simulink model "boost_converter_example"  (R2025a)
settings: Solver=FixedStepAuto  StartTime=0.0  StopTime=Tfin  FixedStep=Ts  RelTol=1e-3
values from neighbouring files (symbols this model uses):
  static_gain = 1.76    [experiment_setup_simulink.m]
  time_constant = 0.5    [experiment_setup_simulink.m]
  u0 = 0    [experiment_setup_simulink.m]    (also in generare_subiect_norocos_TOATE_2024.m = 30+5*rand(1); ordin1_treapta.m = mean(u(i1:i2)); ordin2_treapta.m = mean(u(i1:i2)))
  ust = 2    [experiment_setup_simulink.m]    (also in generare_subiect_norocos_TOATE_2024.m = u0+20*rand(1); master_tapes_ord2_imp_reg_mod.m = mean(u(i1:i2)); ordin1_treapta.m = mean(u(j1:j2)); ordin2_treapta.m = mean(u(j1:j2)))
  whtn_pow_in = 1e-5    (= 1e-05)    [experiment_setup_simulink.m]
  whtn_pow_out = 1e-6    (= 1e-06)    [experiment_setup_simulink.m]
  whtn_seed_in = 23341    [experiment_setup_simulink.m]
  whtn_seed_out = 23342    [experiment_setup_simulink.m]
  whtn_Ts_in = Ts    (= 0.01)    [experiment_setup_simulink.m]
  whtn_Ts_out = Ts    (= 0.01)    [experiment_setup_simulink.m]
  x0 = -0.5    [experiment_setup_simulink.m]
libraries: simulink x3
settings Model: Creator=mircea  LastModifiedBy=mircea

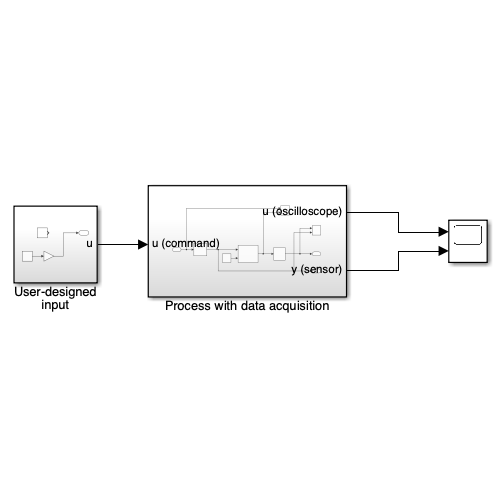
[thumbnail: Simulink's stored preview of the top-level diagram]
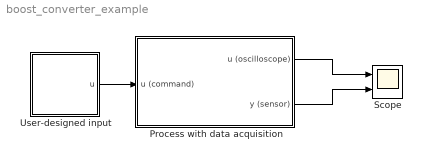
== system boost_converter_example ==
  Process with data acquisition : Subsystem
  Scope : Scope  NumInputPorts=2
      settings: ActiveDisplayYMinimum=-3.990234375  ActiveDisplayYMaximum=5.130859375
  User-designed input : Subsystem
  wires:
  Process with data acquisition/1(u (oscilloscope)) -> Scope/1
  Process with data acquisition/2(y (sensor)) -> Scope/2
  User-designed input/1(u) -> Process with data acquisition/1(u (command))

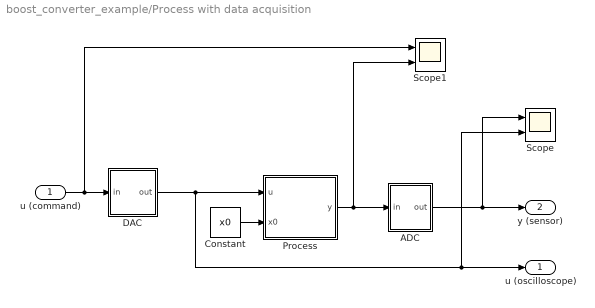
== system boost_converter_example/Process with data acquisition ==
  u (command) : Inport
  ADC : Subsystem
  Constant : Constant  Value=x0
  DAC : Subsystem
  Process : Subsystem
  Scope : Scope  NumInputPorts=2
      settings: ActiveDisplayYMinimum=-1.328125  ActiveDisplayYMaximum=1.328125
  Scope1 : Scope  NumInputPorts=2
      settings: ActiveDisplayYMinimum=-1.328125  ActiveDisplayYMaximum=1.328125  DataLoggingVariableName=ScopeData2
  u (oscilloscope) : Outport
  y (sensor) : Outport  Port=2
  wires:
  Constant/1 -> Process/2(x0)
  u (command)/1 -> Scope1/1, DAC/1(in)
  Process/1(y) -> Scope1/2, ADC/1(in)
  ADC/1(out) -> Scope/1, y (sensor)/1
  DAC/1(out) -> Scope/2, u (oscilloscope)/1, Process/1(u)

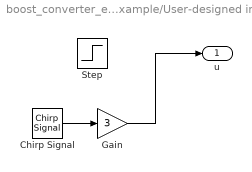
== system boost_converter_example/User-designed input ==
  Chirp Signal : simulink/Sources/Chirp Signal  f1=0.01  T=80  f2=15
  Gain : Gain  Gain=3
  Step : Step  Before=u0  After=ust  SampleTime=0
  u : Outport
  wires:
  Chirp Signal/1 -> Gain/1
  Gain/1 -> u/1

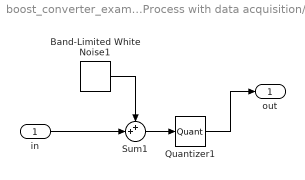
== system boost_converter_example/Process with data acquisition/ADC ==
  in : Inport
  Band-Limited White Noise1 : simulink/Sources/Band-Limited White Noise  Cov=[whtn_pow_out]  Ts=whtn_Ts_out  seed=[whtn_seed_out]
  Quantizer1 : Quantizer  QuantizationInterval=q_out
  Sum1 : Sum  Inputs=++|
  out : Outport
  wires:
  Quantizer1/1 -> out/1
  Sum1/1 -> Quantizer1/1
  in/1 -> Sum1/2
  Band-Limited White Noise1/1 -> Sum1/1

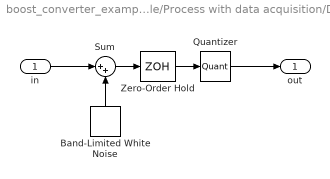
== system boost_converter_example/Process with data acquisition/DAC ==
  in : Inport
  Band-Limited White Noise : simulink/Sources/Band-Limited White Noise  Cov=[whtn_pow_in]  Ts=whtn_Ts_in  seed=[whtn_seed_in]
  Quantizer : Quantizer  QuantizationInterval=q_in
  Sum : Sum  Inputs=|++
  Zero-Order Hold : ZeroOrderHold  SampleTime=-1
  out : Outport
  wires:
  Quantizer/1 -> out/1
  Sum/1 -> Zero-Order Hold/1
  in/1 -> Sum/1
  Band-Limited White Noise/1 -> Sum/2
  Zero-Order Hold/1 -> Quantizer/1

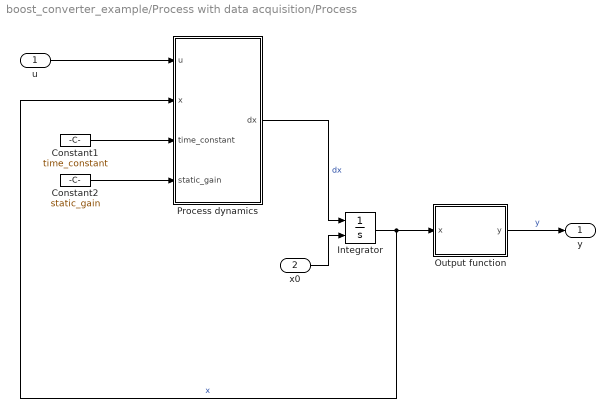
== system boost_converter_example/Process with data acquisition/Process ==
  u : Inport
  x0 : Inport  Port=2
  Constant1 : Constant  Value=time_constant
  Constant2 : Constant  Value=static_gain
  Integrator : Integrator  InitialConditionSource=external
  Output function : MATLAB Function  TreatAsAtomicUnit=on
  Process dynamics : MATLAB Function  TreatAsAtomicUnit=on
  y : Outport
  wires:
  u/1 -> Process dynamics/1(u)
  Process dynamics/1(dx) -> Integrator/1  "dx"
  Integrator/1 -> Output function/1(x), Process dynamics/2(x)  "x"
  Output function/1(y) -> y/1  "y"
  x0/1 -> Integrator/2
  Constant2/1 -> Process dynamics/4(static_gain)
  Constant1/1 -> Process dynamics/3(time_constant)

== matlab function boost_converter_example/Process with data acquisition/Process/Process dynamics ==
  data: u input; dx output; x input; time_constant input; static_gain input
function dx = fcn(u,x,time_constant,static_gain)
dx = -1/time_constant*x + static_gain/time_constant*u;

== matlab function boost_converter_example/Process with data acquisition/Process/Output function ==
  data: y output; x input
function y = fcn(x)

y = x;

end
